simulink model "outmodc_mdl"  (R2021b)
settings: Solver=ode1  StartTime=0.0  StopTime=140  FixedStep=0.0001  MaxStep=0.1  MinStep=0.01  RelTol=1e-3
values from neighbouring files (symbols this model uses):
  A = [0 1; 0 0]    [pendulum_data.m]
  Am = A+B*Lx    [obsmod_data.m]    (also in outmod_data.m; outmodc_data.m; stmod_data.m = A+B*F)
  B = [0;1]    [pendulum_data.m]
  Bm = B*-inv(Cm*inv(Am)*B)    [obsmod_data.m]    (also in outmod_data.m; outmodc_data.m; stmod_data.m = B*G)
  C = C([1,3],:)    [comp_data.m]    (also in pendulum_data.m = [1 1])
  L = -inv(S*B)*(S*Am-Phi*S)    [stmod_data.m]
  rho = 1    [comp_data.m]    (also in obsint_data.m; obsmod_data.m; outmod_data.m; outmodc_data.m)
  S = rpp(A,B,psm)    [obsint_data.m]    (also in stint_data.m = rpp(A,B,sp); stmod_data.m = inv(S*B)*S; streg_data.m = rpp(A,B,sp))
  x0 = zeros(1,n)    [comp_data.m]    (also in obsint_data.m; obsmod_data.m; outmod_data.m; outmodc_data.m)
  z0 = zeros(1,n)    [obsint_data.m]    (also in obsmod_data.m; pendulum_data.m)
undefined symbols (not defined in the file or in its folder): Dhat, Hhat, Lam, Lr, Lx, m, n, P, p
settings Model: Creator=w.schwamm  LastModifiedBy=w.schwamm
settings DataIOCC: SaveOutput=off  SaveTime=off  ReturnWorkspaceOutputs=off  StateSaveName=x  TimeSaveName=t  OutputSaveName=y

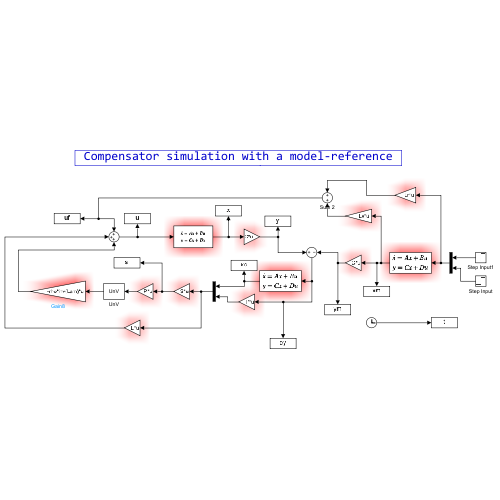
[thumbnail: Simulink's stored preview of the top-level diagram]
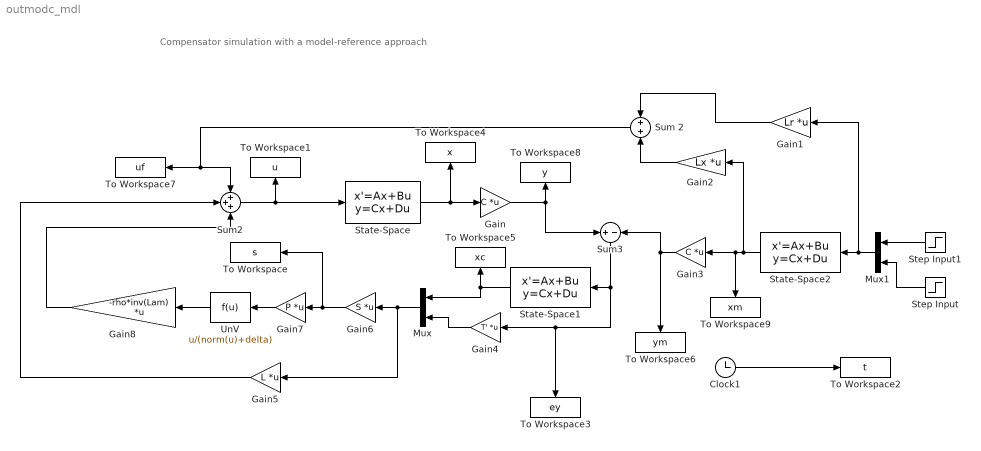
== system outmodc_mdl ==
  note: Compensator simulation with a model-reference approach
  Clock1 : Clock
  Gain : Gain  Gain=C  Multiplication=Matrix(K*u)
  Gain1 : Gain  Gain=Lr  Multiplication=Matrix(K*u)
  Gain2 : Gain  Gain=Lx  Multiplication=Matrix(K*u)
  Gain3 : Gain  Gain=C  Multiplication=Matrix(K*u)
  Gain4 : Gain  Gain=T'  Multiplication=Matrix(K*u)
  Gain5 : Gain  Gain=L  Multiplication=Matrix(K*u)
  Gain6 : Gain  Gain=S  Multiplication=Matrix(K*u)
  Gain7 : Gain  Gain=P  Multiplication=Matrix(K*u)
  Gain8 : Gain  Gain=-rho*inv(Lam)  Multiplication=Matrix(K*u)
  Mux : Mux  Inputs=2
  Mux1 : Mux  Inputs=2
  State-Space : StateSpace  A=A  B=B  C=eye(n)  D=zeros(n,m)  InitialCondition=x0
  State-Space1 : StateSpace  A=Hhat  B=Dhat  C=eye(n-p)  D=zeros(n-p,p)  InitialCondition=z0
  State-Space2 : StateSpace  A=Am  B=Bm  C=eye(n)  D=zeros(n,m)  InitialCondition=0
  Step Input : Step  Time=0  After=0  SampleTime=0
  Step Input1 : Step  Time=0  After=0.25  SampleTime=0
  Sum 2 : Sum
  Sum2 : Sum  Inputs=+++
  Sum3 : Sum  Inputs=+-
  To Workspace : ToWorkspace  VariableName=s  SaveFormat=Timeseries  SampleTime=-1
      settings: MaxDataPoints=1000000
  To Workspace1 : ToWorkspace  VariableName=u  SaveFormat=Timeseries  SampleTime=-1
      settings: MaxDataPoints=1000000
  To Workspace2 : ToWorkspace  VariableName=t  SaveFormat=Timeseries  SampleTime=-1
      settings: MaxDataPoints=1000000
  To Workspace3 : ToWorkspace  VariableName=ey  SaveFormat=Timeseries  SampleTime=-1
      settings: MaxDataPoints=1000000
  To Workspace4 : ToWorkspace  VariableName=x  SaveFormat=Timeseries  SampleTime=-1
      settings: MaxDataPoints=1000000
  To Workspace5 : ToWorkspace  VariableName=xc  SaveFormat=Timeseries  SampleTime=-1
      settings: MaxDataPoints=1000000
  To Workspace6 : ToWorkspace  VariableName=ym  SaveFormat=Timeseries  SampleTime=-1
      settings: MaxDataPoints=1000000
  To Workspace7 : ToWorkspace  VariableName=uf  SaveFormat=Timeseries  SampleTime=-1
      settings: MaxDataPoints=1000000
  To Workspace8 : ToWorkspace  VariableName=y  SaveFormat=Timeseries  SampleTime=-1
      settings: MaxDataPoints=1000000
  To Workspace9 : ToWorkspace  VariableName=xm  SaveFormat=Timeseries  SampleTime=-1
      settings: MaxDataPoints=1000000
  UnV : Fcn  Expr=u/(norm(u)+delta)  mask(unit vector){delta=0.01}
      mask Display: disp('UnV')
  wires:
  State-Space/1 -> Gain/1, To Workspace4/1
  Clock1/1 -> To Workspace2/1
  Sum2/1 -> To Workspace1/1, State-Space/1
  Gain5/1 -> Sum2/2
  State-Space2/1 -> Gain2/1, Gain3/1, To Workspace9/1
  Gain/1 -> Sum3/1, To Workspace8/1
  Gain3/1 -> Sum3/2, To Workspace6/1
  Sum3/1 -> State-Space1/1, Gain4/1, To Workspace3/1
  Sum 2/1 -> Sum2/1, To Workspace7/1
  UnV/1 -> Gain8/1
  Gain8/1 -> Sum2/3
  Step Input1/1 -> Mux1/1
  Mux/1 -> Gain6/1, Gain5/1
  Gain4/1 -> Mux/2
  State-Space1/1 -> Mux/1, To Workspace5/1
  Gain6/1 -> Gain7/1, To Workspace/1
  Gain7/1 -> UnV/1
  Mux1/1 -> Gain1/1, State-Space2/1
  Step Input/1 -> Mux1/2
  Gain1/1 -> Sum 2/1
  Gain2/1 -> Sum 2/2
